simulink model "UltrasoundEnhancementSubsystem"  (R2024b)
settings: Solver=FixedStepAuto  StartTime=0  StopTime=0  FixedStep=1  RelTol=1e-3
settings Model: Creator=rohit  LastModifiedBy=rohit

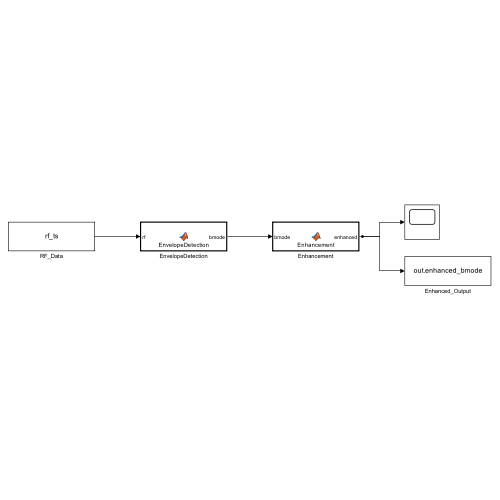
[thumbnail: Simulink's stored preview of the top-level diagram]
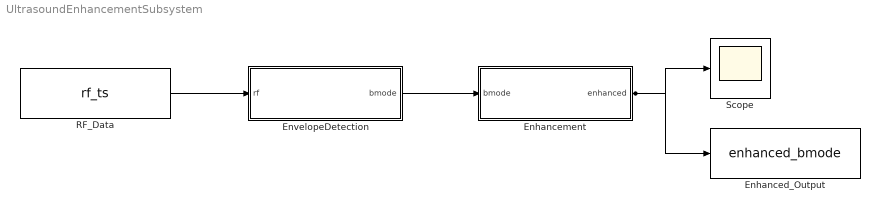
== system UltrasoundEnhancementSubsystem ==
  Enhanced_Output : ToWorkspace  VariableName=enhanced_bmode  SampleTime=-1
  Enhancement : MATLAB Function  TreatAsAtomicUnit=on
  EnvelopeDetection : MATLAB Function  TreatAsAtomicUnit=on
  RF_Data : FromWorkspace  VariableName=rf_ts
  Scope : Scope
  wires:
  RF_Data/1 -> EnvelopeDetection/1(rf)
  EnvelopeDetection/1(bmode) -> Enhancement/1(bmode)
  Enhancement/1(enhanced) -> Scope/1, Enhanced_Output/1

== matlab function UltrasoundEnhancementSubsystem/EnvelopeDetection ==
  data: rf input; bmode output
function bmode = EnvelopeDetection(rf)
% Envelope detection on raw RF data
% Input:  rf     - [num_samples x num_elements] raw RF matrix
% Output: bmode  - [num_samples x num_elements] log-compressed B-mode image

[num_samples, num_elements] = size(rf);
bmode = zeros(num_samples, num_elements);

for col = 1:num_elements
    env = abs(hilbert(rf(:, col)));
    env(env < 1e-6) = 1e-6;
    bmode(:, col) = 20 * log10(env);
end

% Normalise to 0-1 range (clip noise floor)
bmode = bmode - max(bmode(:));
bmode = max(bmode, -60);
bmode = (bmode + 60) / 60;

== matlab function UltrasoundEnhancementSubsystem/Enhancement ==
  data: bmode input; enhanced output
function enhanced = Enhancement(bmode)
% Median filter enhancement on log-compressed B-mode image
% Input:  bmode    - [num_samples x num_elements] normalised B-mode (0 to 1)
% Output: enhanced - [num_samples x num_elements] median-filtered image (0-255)

% Apply 3x3 median filter (matches Phase 3 selection: PSNR 24.77 dB, SSIM 0.4011)
filtered = medfilt2(bmode, [3 3]);

% Scale to 0-255 for CNN input compatibility
enhanced = filtered * 255;
